simulink library "vmc"  (R2021b)
settings: Solver=VariableStepAuto  StartTime=0.0  StopTime=10.0  RelTol=1e-3
undefined symbols (not defined in the file or in its folder): AVMC_ACCDeltaTqIGain_X_kph, AVMC_ACCDeltaTqIGain_Y_mps2, AVMC_ACCDeltaTqIGainP2_X_kph, AVMC_ACCDeltaTqIGainP2_Y_mps2, AVMC_ACCDeltaTqPGain_X_kph, AVMC_ACCDeltaTqPGain_Y_kph, AVMC_ACCDeltaTqPGainP2_X_kph, AVMC_ACCDeltaTqPGainP2_Y_kph, AVMC_ACCLongSteadyCtrl_X_kph, AVMC_CCAccelCMD_X_kph, AVMC_CCAccelCMD_Y_kph, AVMC_CCDeltaTqIGain_X_kph, AVMC_CCDeltaTqIGain_Y_mps2, AVMC_CCDeltaTqPGain_X_kph, AVMC_CCDeltaTqPGain_Y_kph, AVMC_CCLongSteadyCtrl_X_kph, AVMC_DISCDeltaTqIGainP2_X_kph, AVMC_DISCDeltaTqIGainP2_Y_mps2, AVMC_ESCRegenOut_X_kph, AVMC_ESCRegenOut_Y_Deg, AVMC_ESCRegenOutEnSpd_X_Deg, AVMC_LatESCRegenOut_X_kph, AVMC_LatESCRegenOut_Y_Deg, AVMC_LongAccDeadZone_X_kph, AVMC_LongAccDeadZoneP2_X_kph, AVMC_LongAccFiltTs_X_Gps, AVMC_LongAccFiltTsP2_X_Gps, AVMC_MCPresBaseTq_X_bar, AVMC_MSAAccelCMD_X_kph, AVMC_MSAAccelCMD_Y_kph, AVMC_MSADeltaTqIGain_X_kph, AVMC_MSADeltaTqIGain_Y_mps2, AVMC_MSADeltaTqPGain_X_kph, AVMC_MSADeltaTqPGain_Y_kph, AVMC_MSALongSteadyCtrl_X_kph, AVMC_MSAPedalOvrd_X_kph, AVMC_MSASpdBand_X_kph, AVMC_OPDDisSlideRate_X_Deg, AVMC_RDCDetectTime_X_kph, AVMC_RDCDetectTime_Y_pct, AVMC_RDCEnSlideRate_X_Deg, AVMC_StESCYaw_X_kph, AVMC_StESCYaw_Y_Deg, AVMC_StESCYawCom_X_kph, AVMC_StESCYawCom_Y_Gps, AVMC_TMSpdBaseTq_X_rpm, C_TASK_10MS_S, C_TASK_5MS_S, DEG2RAD, Discrete, ENUM_ADASACCSTA_ACTIVE, ENUM_ADASACCSTA_OVERRIDE, ENUM_ADASACCSTA_STANDBY, ENUM_ADASMSASTA_ACTIVE, ENUM_ADASMSASTA_ERROR, ENUM_ADASMSASTA_OFF, ENUM_ADASMSASTA_OVERSPEED, ENUM_ADASMSASTA_STANDBY, ENUM_ADASMSASTA_UNDERSPEED, ENUM_ADASMSASTA_UNLIMIT ... (+254)
libraries: hcu_lib x57, simulink x49, ctrlSharedLib x6, simulink_extras x1
(part 6 of 9)

== system vmc/VMC/Slide Rate  Calculation/4Wheel Calculation ==
  VINP_LFRawWhlSpeed_kph : Inport
  VINP_RFRawWhlSpeed_kph : Inport  Port=2
  VINP_LRRawWhlSpeed_kph : Inport  Port=3
  VINP_RRRawWhlSpeed_kph : Inport  Port=4
  VVMC_LongAcc_Gps : Inport  Port=5
  task_time_s : Inport  Port=6
  VINP_VehSpeed_kph : Inport  Port=7
  VTQD_AfterAvailableTqDemFr_Nm : Inport  Port=8
  VTQD_AfterAvailableTqDemRr_Nm : Inport  Port=9
  VTQD_GearActualPosn_enum : Inport  Port=10
  VINP_LongAccel_Gps : Inport  Port=11
  VVMC_CalibratedAccX_G : Inport  Port=12
  Constant1 : Constant  Value=KVMC_SlideRateLongGSW_flg
  Constant3 : Constant  Value=KVMC_4WheelLongAccSW_flg
  Determination : Subsystem
  LF Wheel : Subsystem
  LR Wheel : Subsystem
  RF Wheel : Subsystem
  RR Wheel : Subsystem
  Switch : Switch  Criteria=u2 > Threshold
  Switch1 : Switch  Criteria=u2 > Threshold
  VVMC_LF4WhlSpdSlideRate_pct : Outport
  VVMC_RF4WhlSpdSlideRate_pct : Outport  Port=2
  VVMC_LR4WhlSpdSlideRate_pct : Outport  Port=3
  VVMC_RR4WhlSpdSlideRate_pct : Outport  Port=4
  VVMC_PredictVehSpd_kph : Outport  Port=5
  VVMC_4WhlSpdSlideRate_pct : Outport  Port=6
  VVMC_AllWhlSkid_flg : Outport  Port=7
  wires:
  [VVMC_4WhlSpdSlideRate_pct] -> VVMC_4WhlSpdSlideRate_pct/1
  [VVMC_PredictVehSpd_kph] -> VVMC_PredictVehSpd_kph/1
  VINP_VehSpeed_kph/1 -> [VINP_VehSpeed_kph]
  task_time_s/1 -> [task_time_s]
  [VVMC_LR4WhlSpdSlideRate_pct] -> VVMC_LR4WhlSpdSlideRate_pct/1
  [VVMC_RR4WhlSpdSlideRate_pct] -> VVMC_RR4WhlSpdSlideRate_pct/1
  [VVMC_RF4WhlSpdSlideRate_pct] -> VVMC_RF4WhlSpdSlideRate_pct/1
  [VVMC_LF4WhlSpdSlideRate_pct] -> VVMC_LF4WhlSpdSlideRate_pct/1
  VINP_LRRawWhlSpeed_kph/1 -> [VINP_LRRawWhlSpeed_kph]
  VINP_LFRawWhlSpeed_kph/1 -> [VINP_LFRawWhlSpeed_kph]
  VINP_RFRawWhlSpeed_kph/1 -> [VINP_RFRawWhlSpeed_kph]
  VINP_RRRawWhlSpeed_kph/1 -> [VINP_RRRawWhlSpeed_kph]
  [VVMC_AllWhlSkid_flg] -> VVMC_AllWhlSkid_flg/1
  VTQD_AfterAvailableTqDemFr_Nm/1 -> [VTQD_AfterAvailableTqDemFr_Nm]
  VTQD_AfterAvailableTqDemRr_Nm/1 -> [VTQD_AfterAvailableTqDemRr_Nm]
  VTQD_GearActualPosn_enum/1 -> [VTQD_GearActualPosn_enum]
  [VVMC_LRPreVehSpd_kph] -> Determination/17(VVMC_LRPreVehSpd_kph)
  [VVMC_4WheelLongAcc_Gps] -> LF Wheel/1(VVMC_4WheelLongAcc_Gps)
  [VINP_RRRawWhlSpeed_kph] -> RR Wheel/3(VINP_RRRawWhlSpeed_kph)
  [VINP_LRRawWhlSpeed_kph] -> LR Wheel/3(VINP_LRRawWhlSpeed_kph)
  [VINP_RFRawWhlSpeed_kph] -> RF Wheel/3(VINP_RFRawWhlSpeed_kph)
  [VTQD_GearActualPosn_enum] -> RF Wheel/4(VTQD_GearActualPosn_enum)
  LF Wheel/1(VVMC_LFPreVehSpd_kph) -> [VVMC_LFPreVehSpd_kph]
  RR Wheel/1(VVMC_RRPreVehSpd_kph) -> [VVMC_RRPreVehSpd_kph]
  [VTQD_GearActualPosn_enum] -> LR Wheel/4(VTQD_GearActualPosn_enum)
  [VVMC_LF4WhlSpdSlideRate_pct] -> Determination/9(VVMC_LF4WhlSpdSlideRate_pct)
  [VVMC_RRWhlSkid_flg] -> Determination/8(VVMC_RRWhlSkid_flg)
  [VINP_LFRawWhlSpeed_kph] -> LF Wheel/3(VINP_LFRawWhlSpeed_kph)
  [task_time_s] -> RR Wheel/2(task_time_s)
  [task_time_s] -> RF Wheel/2(task_time_s)
  [VVMC_RR4WhlSpdSlideRate_pct] -> Determination/12(VVMC_RR4WhlSpdSlideRate_pct)
  RR Wheel/3(VVMC_RR4WhlSpdSlideRate_pct) -> [VVMC_RR4WhlSpdSlideRate_pct]
  [VTQD_AfterAvailableTqDemFr_Nm] -> Determination/13(VTQD_AfterAvailableTqDemFr_Nm)
  [VVMC_LR4WhlSpdSlideRate_pct] -> Determination/11(VVMC_LR4WhlSpdSlideRate_pct)
  [VTQD_GearActualPosn_enum] -> Determination/4(VTQD_GearActualPosn_enum)
  [task_time_s] -> Determination/2(task_time_s)
  [VVMC_LFWhlSkid_flg] -> Determination/5(VVMC_LFWhlSkid_flg)
  [VINP_VehSpeed_kph] -> Determination/3(VINP_VehSpeed_kph)
  [VVMC_RRPreVehSpd_kph] -> Determination/18(VVMC_RRPreVehSpd_kph)
  Determination/2(VVMC_AllWhlSkid_flg) -> [VVMC_AllWhlSkid_flg]
  Determination/1(VVMC_PredictVehSpd_kph) -> [VVMC_PredictVehSpd_kph]
  Determination/3(VVMC_4WhlSpdSlideRate_pct) -> [VVMC_4WhlSpdSlideRate_pct]
  [VVMC_RFWhlSkid_flg] -> Determination/6(VVMC_RFWhlSkid_flg)
  LR Wheel/3(VVMC_LR4WhlSpdSlideRate_pct) -> [VVMC_LR4WhlSpdSlideRate_pct]
  LR Wheel/2(VVMC_LRWhlSkid_flg) -> [VVMC_LRWhlSkid_flg]
  [VVMC_LRWhlSkid_flg] -> Determination/7(VVMC_LRWhlSkid_flg)
  RF Wheel/1(VVMC_RFPreVehSpd_kph) -> [VVMC_RFPreVehSpd_kph]
  [task_time_s] -> LR Wheel/2(task_time_s)
  [VVMC_RFPreVehSpd_kph] -> Determination/16(VVMC_RFPreVehSpd_kph)
  LR Wheel/1(VVMC_LRPreVehSpd_kph) -> [VVMC_LRPreVehSpd_kph]
  [VVMC_4WheelLongAcc_Gps] -> RF Wheel/1(VVMC_4WheelLongAcc_Gps)
  RR Wheel/2(VVMC_RRWhlSkid_flg) -> [VVMC_RRWhlSkid_flg]
  [VVMC_LFPreVehSpd_kph] -> Determination/15(VVMC_LFPreVehSpd_kph)
  [VVMC_RF4WhlSpdSlideRate_pct] -> Determination/10(VVMC_RF4WhlSpdSlideRate_pct)
  [VTQD_AfterAvailableTqDemRr_Nm] -> Determination/14(VTQD_AfterAvailableTqDemRr_Nm)
  LF Wheel/2(VVMC_LFWhlSkid_flg) -> [VVMC_LFWhlSkid_flg]
  RF Wheel/2(VVMC_RFWhlSkid_flg) -> [VVMC_RFWhlSkid_flg]
  [VVMC_4WheelLongAcc_Gps] -> Determination/1(VVMC_4WheelLongAcc_Gps)
  [VVMC_4WheelLongAcc_Gps] -> RR Wheel/1(VVMC_4WheelLongAcc_Gps)
  [VTQD_GearActualPosn_enum] -> RR Wheel/4(VTQD_GearActualPosn_enum)
  [VVMC_4WheelLongAcc_Gps] -> LR Wheel/1(VVMC_4WheelLongAcc_Gps)
  RF Wheel/3(VVMC_RF4WhlSpdSlideRate_pct) -> [VVMC_RF4WhlSpdSlideRate_pct]
  LF Wheel/3(VVMC_LF4WhlSpdSlideRate_pct) -> [VVMC_LF4WhlSpdSlideRate_pct]
  [task_time_s] -> LF Wheel/2(task_time_s)
  [VTQD_GearActualPosn_enum] -> LF Wheel/4(VTQD_GearActualPosn_enum)
  Constant3/1 -> Switch/2
  Switch/1 -> [VVMC_4WheelLongAcc_Gps]  "VVMC_4WheelLongAcc_Gps"
  VINP_LongAccel_Gps/1 -> [VINP_LongAccel_Gps]
  VVMC_LongAcc_Gps/1 -> [VVMC_LongAcc_Gps]
  [VVMC_LongAcc_Gps] -> Switch/3
  Switch1/1 -> Switch/1
  [VINP_LongAccel_Gps] -> Switch1/3
  Constant1/1 -> Switch1/2
  [VVMC_CalibratedAccX_G] -> Switch1/1
  VVMC_CalibratedAccX_G/1 -> [VVMC_CalibratedAccX_G]

== system vmc/VMC/Slide Rate  Calculation/Alternative Wheel Slide Calculation ==
  VINP_LFRawWhlSpeed_kph : Inport
  VINP_RFRawWhlSpeed_kph : Inport  Port=2
  VINP_LRRawWhlSpeed_kph : Inport  Port=3
  VINP_RRRawWhlSpeed_kph : Inport  Port=4
  Abs : Abs
  Abs1 : Abs
  Add : Sum  Inputs=+-
  Add1 : Sum  Inputs=+-
  Constant{,3,5,8} (4 alike) : Constant  Value=KVMC_RawWhlSpeedDeadZone_kph
  Constant1 : Constant  Value=ONE_FLOAT
  Constant2 : Constant  Value=ONE_PERCENT
  Constant4 : Constant  Value=ZERO_FLOAT
  Constant6 : Constant  Value=ONE_FLOAT
  Constant7 : Constant  Value=ONE_PERCENT
  Constant9 : Constant  Value=ZERO_FLOAT
  Divide : Product  Inputs=*//
  Divide1 : Product  Inputs=*//
  Relational Operator{,1..3} (4 alike) : RelationalOperator  Operator=<=  OutDataTypeStr=boolean  RndMeth=Simplest
  Relational Operator4 : RelationalOperator  OutDataTypeStr=boolean  RndMeth=Simplest
  Switch{,1..4} (5 alike) : Switch  Criteria=u2 > Threshold
  VVMC_AltLWhlSlideRate_pct : Outport
  VVMC_AltRWhlSlideRate_pct : Outport  Port=2
  VVMC_AltWhlSlideRate_pct : Outport  Port=3
  wires:
  VINP_RRRawWhlSpeed_kph/1 -> [VINP_RRRawWhlSpeed_kph]
  Relational Operator1/1 -> Switch1/2
  Abs/1 -> Relational Operator4/1
  Divide/1 -> Switch1/3  "VVMC_CalAltLWhlSlideRate_pct"
  Constant1/1 -> Switch/1
  [VINP_LFRawWhlSpeed_kph] -> Add/2
  Switch1/1 -> [VVMC_AltLWhlSlideRate_pct]  "VVMC_AltLWhlSlideRate_pct"
  Constant6/1 -> Switch2/1
  Relational Operator3/1 -> Switch3/2
  Relational Operator4/1 -> Switch4/2
  [VVMC_AltLWhlSlideRate_pct] -> Abs/1
  [VVMC_AltLWhlSlideRate_pct] -> VVMC_AltLWhlSlideRate_pct/1
  VINP_LFRawWhlSpeed_kph/1 -> [VINP_LFRawWhlSpeed_kph]
  VINP_LRRawWhlSpeed_kph/1 -> [VINP_LRRawWhlSpeed_kph]
  VINP_RFRawWhlSpeed_kph/1 -> [VINP_RFRawWhlSpeed_kph]
  [VVMC_AltRWhlSlideRate_pct] -> Switch4/3
  Switch3/1 -> [VVMC_AltRWhlSlideRate_pct]  "VVMC_AltRWhlSlideRate_pct"
  Constant4/1 -> Switch1/1
  Constant3/1 -> Relational Operator1/2
  [VVMC_AltRWhlSlideRate_pct] -> Abs1/1
  [VVMC_AltLWhlSlideRate_pct] -> Switch4/1
  Switch4/1 -> [VVMC_AltWhlSlideRate_pct]  "VVMC_AltWhlSlideRate_pct"
  Constant2/1 -> Divide/2
  Constant7/1 -> Divide1/2
  Switch/1 -> Divide/3
  Constant9/1 -> Switch3/1
  [VINP_LFRawWhlSpeed_kph] -> Switch/3
  Relational Operator/1 -> Switch/2
  [VVMC_AltWhlSlideRate_pct] -> VVMC_AltWhlSlideRate_pct/1
  [VINP_RFRawWhlSpeed_kph] -> Add1/2
  Add/1 -> Divide/1
  Constant/1 -> Relational Operator/2
  [VINP_LFRawWhlSpeed_kph] -> Relational Operator1/1
  Abs1/1 -> Relational Operator4/2
  [VINP_RRRawWhlSpeed_kph] -> Add1/1
  [VINP_RFRawWhlSpeed_kph] -> Relational Operator3/1
  [VINP_RFRawWhlSpeed_kph] -> Switch2/3
  Add1/1 -> Divide1/1
  [VINP_LFRawWhlSpeed_kph] -> Relational Operator/1
  [VINP_LRRawWhlSpeed_kph] -> Add/1
  [VINP_RFRawWhlSpeed_kph] -> Relational Operator2/1
  Constant8/1 -> Relational Operator3/2
  Constant5/1 -> Relational Operator2/2
  Divide1/1 -> Switch3/3  "VVMC_CalAltRWhlSlideRate_pct"
  Switch2/1 -> Divide1/3
  Relational Operator2/1 -> Switch2/2
  [VVMC_AltRWhlSlideRate_pct] -> VVMC_AltRWhlSlideRate_pct/1

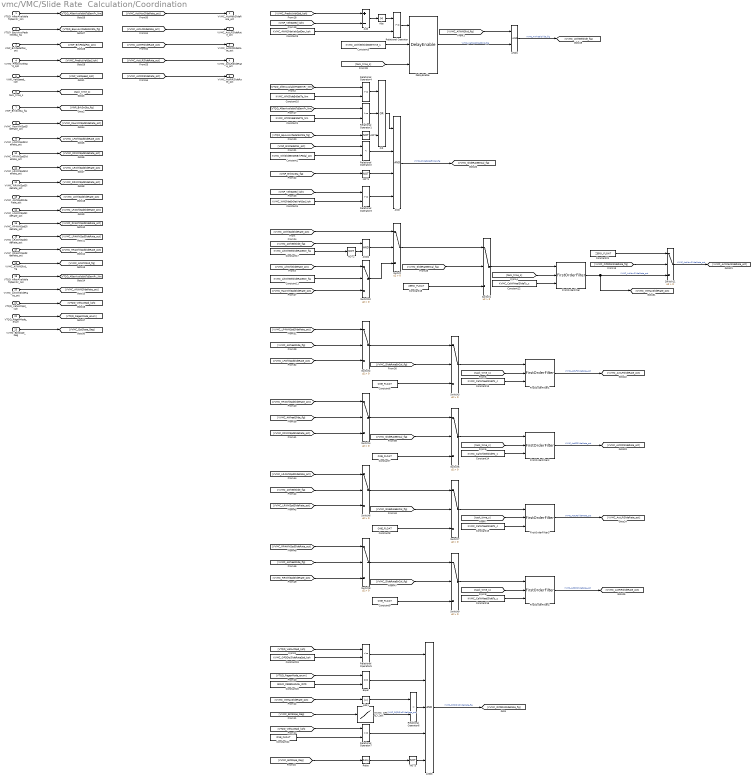
== system vmc/VMC/Slide Rate  Calculation/Coordination ==
  VTQD_AfterAvailableTqDemFr_Nm : Inport
  VTQD_EquivAccPedalSWSta_flg : Inport  Port=2
  VINP_BrkPedalPos_pct : Inport  Port=3
  VVMC_PredictVehSpd_kph : Inport  Port=4
  VINP_VehSpeed_kph : Inport  Port=5
  task_time_s : Inport  Port=6
  VINP_BrkSwSta_flg : Inport  Port=7
  VVMC_RawWhlSpdSlideRate_pct : Inport  Port=8
  VVMC_LFWhlSpdSlideRate_pct : Inport  Port=9
  VVMC_RFWhlSpdSlideRate_pct : Inport  Port=10
  VVMC_LRWhlSpdSlideRate_pct : Inport  Port=11
  VVMC_RRWhlSpdSlideRate_pct : Inport  Port=12
  VVMC_4WhlSpdSlideRate_pct : Inport  Port=13
  VVMC_LF4WhlSpdSlideRate_pct : Inport  Port=14
  VVMC_RF4WhlSpdSlideRate_pct : Inport  Port=15
  VVMC_LR4WhlSpdSlideRate_pct : Inport  Port=16
  VVMC_RR4WhlSpdSlideRate_pct : Inport  Port=17
  VVMC_AllWhlSkid_flg : Inport  Port=18
  VTQD_AfterAvailableTqDemRr_Nm : Inport  Port=19
  VVMC_AltWhlSlideRate_pct : Inport  Port=20
  VTQD_VehActSpd_kph : Inport  Port=21
  VTQD_RegenMode_enum : Inport  Port=22
  VVMC_EstSlope_Deg : Inport  Port=23
  AND : Logic  Inputs=4  AllPortsSameDT=off  OutDataTypeStr=boolean
  AND1 : Logic  AllPortsSameDT=off  OutDataTypeStr=boolean
  AND2 : Logic  AllPortsSameDT=off  OutDataTypeStr=boolean
  AND3 : Logic  Inputs=5  AllPortsSameDT=off  OutDataTypeStr=boolean
  Abs : Abs
  Abs1 : Abs
  Add : Sum  Inputs=+-
  Constant1 : Constant  Value=KVMC_WhlSlideEnDetTq_Nm
  Constant10 : Constant  Value=KVMC_WhlSlideEnDetTq_Nm
  Constant11 : Constant  Value=KVMC_AltWheelSlideRateSW_flg
  Constant{12..16} (5 alike) : Constant  Value=KVMC_CalWhleelSlideTs_c
  Constant17 : Constant  Value=KVMC_AltWheelSlideRateSW_flg
  Constant18 : Constant  Value=ZERO_FLOAT
  Constant19 : Constant  Value=KVMC_OPDDisSlideRateSpd_kph
  Constant2 : Constant  Value=KVMC_WhlSlideEnDetBrkPedal_pct
  Constant20 : Constant  Value=ENUM_REGENLEVEL_OPD
  Constant21 : Constant  Value=ZERO_FLOAT
  Constant{6..9,22} (5 alike) : Constant  Value=ONE_FLOAT
  Constant3 : Constant  Value=KVMC_4WhlSlideVehSpdDev_kph
  Constant4 : Constant  Value=KVMC_WhlSlideEnDetVehSpd_kph
  Constant5 : Constant  Value=KVMC_4WhleelSlideDetTime_s
  DelayEnable : hcu_lib/Basic_Blocks/DelayEnable
  Equal : RelationalOperator  Operator===  OutDataTypeStr=boolean  RndMeth=Simplest
  FirstOrderFilter{,1..4} (5 alike) : hcu_lib/Basic_Blocks/FirstOrderFilter
  MVMC_OPDDisSlideRate_Y_pct : Lookup_n-D  NumberOfTableDimensions=1  BreakpointsForDimension1=AVMC_OPDDisSlideRate_X_Deg  Table=MVMC_OPDDisSlideRate_Y_pct  InternalRulePriority=Speed  RndMeth=Simplest  InputSameDT=on
  NOT{,1..3} (4 alike) : Logic  Operator=NOT  AllPortsSameDT=off  OutDataTypeStr=boolean
  OR : Logic  Operator=OR  Inputs=3  AllPortsSameDT=off  OutDataTypeStr=boolean
  Relational Operator{,1,3..4,7} (5 alike) : RelationalOperator  OutDataTypeStr=boolean  RndMeth=Simplest
  Relational Operator2 : RelationalOperator  Operator=<  OutDataTypeStr=boolean  RndMeth=Simplest
  Relational Operator5 : RelationalOperator  Operator=<=  OutDataTypeStr=boolean  RndMeth=Simplest
  Relational Operator6 : RelationalOperator  Operator=<  OutDataTypeStr=boolean  RndMeth=Simplest
  Relay : Relay  OnSwitchValue=KTQD_OPDHoldGradeUp_Deg  OffSwitchValue=KTQD_OPDHoldGradeDown_Deg  OutDataTypeStr=boolean
  Switch{,1..11} (12 alike) : Switch  Criteria=u2 > Threshold
  VVMC_ActMaxSlideRate_pct : Outport
  VVMC_ActLFSlideRate_pct : Outport  Port=2
  VVMC_ActRFSlideRate_pct : Outport  Port=3
  VVMC_ActLRSlideRate_pct : Outport  Port=4
  VVMC_ActRRSlideRate_pct : Outport  Port=5
  wires:
  VVMC_RR4WhlSpdSlideRate_pct/1 -> [VVMC_RR4WhlSpdSlideRate_pct]
  VVMC_LR4WhlSpdSlideRate_pct/1 -> [VVMC_LR4WhlSpdSlideRate_pct]
  VVMC_RF4WhlSpdSlideRate_pct/1 -> [VVMC_RF4WhlSpdSlideRate_pct]
  VVMC_LF4WhlSpdSlideRate_pct/1 -> [VVMC_LF4WhlSpdSlideRate_pct]
  VVMC_4WhlSpdSlideRate_pct/1 -> [VVMC_4WhlSpdSlideRate_pct]
  VVMC_LRWhlSpdSlideRate_pct/1 -> [VVMC_LRWhlSpdSlideRate_pct]
  VVMC_RRWhlSpdSlideRate_pct/1 -> [VVMC_RRWhlSpdSlideRate_pct]
  VVMC_LFWhlSpdSlideRate_pct/1 -> [VVMC_LFWhlSpdSlideRate_pct]
  VVMC_RFWhlSpdSlideRate_pct/1 -> [VVMC_RFWhlSpdSlideRate_pct]
  VVMC_RawWhlSpdSlideRate_pct/1 -> [VVMC_RawWhlSpdSlideRate_pct]
  task_time_s/1 -> [task_time_s]
  VINP_BrkSwSta_flg/1 -> [VINP_BrkSwSta_flg]
  VINP_VehSpeed_kph/1 -> [VINP_VehSpeed_kph]
  VINP_BrkPedalPos_pct/1 -> [VINP_BrkPedalPos_pct]
  VTQD_EquivAccPedalSWSta_flg/1 -> [VTQD_EquivAccPedalSWSta_flg]
  VTQD_AfterAvailableTqDemFr_Nm/1 -> [VTQD_AfterAvailableTqDemFr_Nm]
  VVMC_PredictVehSpd_kph/1 -> [VVMC_PredictVehSpd_kph]
  [VVMC_ActRFSlideRate_pct] -> VVMC_ActRFSlideRate_pct/1
  [VVMC_ActLFSlideRate_pct] -> VVMC_ActLFSlideRate_pct/1
  [VVMC_ActMaxSlideRate_pct] -> VVMC_ActMaxSlideRate_pct/1
  [VVMC_ActLRSlideRate_pct] -> VVMC_ActLRSlideRate_pct/1
  [VVMC_ActRRSlideRate_pct] -> VVMC_ActRRSlideRate_pct/1
  [VINP_VehSpeed_kph] -> Add/2
  OR/1 -> AND/1
  [VVMC_RRWhlSpdSlideRate_pct] -> Switch8/3
  Constant4/1 -> Relational Operator3/2
  [VVMC_4WheelSlide_flg] -> AND2/1
  [VVMC_4WhlSpdSlideRate_pct] -> Switch/1
  [VVMC_SlideRateEnCal_flg] -> Switch9/2
  [VVMC_4WheelSlide_flg] -> Switch6/2
  [VVMC_LR4WhlSpdSlideRate_pct] -> Switch6/1
  [VTQD_EquivAccPedalSWSta_flg] -> NOT/1
  Constant8/1 -> Switch7/3
  [VVMC_LF4WhlSpdSlideRate_pct] -> Switch2/1
  Abs/1 -> Relational Operator/1
  Switch8/1 -> Switch9/1
  [VVMC_LRWhlSpdSlideRate_pct] -> Switch6/3
  [VVMC_SlideRateEnCal_flg] -> Switch5/2
  Switch/1 -> Switch1/1
  Constant7/1 -> Switch5/3
  Switch4/1 -> Switch5/1
  Constant9/1 -> Switch9/3
  Constant5/1 -> DelayEnable/2
  [VINP_BrkPedalPos_pct] -> Relational Operator2/1
  Switch6/1 -> Switch7/1
  NOT1/1 -> AND/3
  [VVMC_RFWhlSpdSlideRate_pct] -> Switch4/3
  [VVMC_SlideRateEnCal_flg] -> Switch3/2
  Constant18/1 -> Switch1/3
  Constant6/1 -> Switch3/3
  Switch2/1 -> Switch3/1
  [VVMC_RF4WhlSpdSlideRate_pct] -> Switch4/1
  [VVMC_4WheelSlide_flg] -> Switch4/2
  Add/1 -> Abs/1
  [VVMC_4WheelSlide_flg] -> Switch2/2
  Relational Operator/1 -> DelayEnable/1
  [VVMC_4WheelSlide_flg] -> Switch8/2
  [VVMC_RR4WhlSpdSlideRate_pct] -> Switch8/1
  Relational Operator3/1 -> AND/4
  [VVMC_LFWhlSpdSlideRate_pct] -> Switch2/3
  Constant1/1 -> Relational Operator1/2
  [VVMC_PredictVehSpd_kph] -> Add/1
  [VINP_BrkSwSta_flg] -> NOT1/1
  [VINP_VehSpeed_kph] -> Relational Operator3/1
  Relational Operator2/1 -> AND/2
  AND/1 -> [VVMC_SlideRateEnCal_flg]  "VVMC_SlideRateEnCal_flg"
  [VVMC_SlideRateEnCal_flg] -> Switch7/2
  Constant3/1 -> Relational Operator/2
  Constant2/1 -> Relational Operator2/2
  [task_time_s] -> DelayEnable/3
  VVMC_AllWhlSkid_flg/1 -> [VVMC_AllWhlSkid_flg]
  DelayEnable/1 -> AND1/2  "VVMC_VehSpdPredSkid_flg"
  AND1/1 -> [VVMC_4WheelSlide_flg]  "VVMC_4WheelSlide_flg"
  [VVMC_AllWhlSkid_flg] -> AND1/1
  Constant10/1 -> Relational Operator4/2
  [VTQD_AfterAvailableTqDemRr_Nm] -> Relational Operator4/1
  NOT/1 -> OR/3
  Relational Operator1/1 -> OR/2
  Relational Operator4/1 -> OR/1
  [VTQD_AfterAvailableTqDemFr_Nm] -> Relational Operator1/1
  VTQD_AfterAvailableTqDemRr_Nm/1 -> [VTQD_AfterAvailableTqDemRr_Nm]
  VVMC_AltWhlSlideRate_pct/1 -> [VVMC_AltWhlSlideRate_pct]
  [VVMC_RawWhlSpdSlideRate_pct] -> Switch10/3
  Switch10/1 -> Switch/3
  [VVMC_AltWhlSlideRate_pct] -> Switch10/1
  Constant11/1 -> Switch10/2
  Switch1/1 -> FirstOrderFilter/1
  FirstOrderFilter1/1 -> [VVMC_ActLFSlideRate_pct]  "VVMC_ActLFSlideRate_pct"
  Switch3/1 -> FirstOrderFilter1/1
  Switch5/1 -> FirstOrderFilter2/1
  FirstOrderFilter2/1 -> [VVMC_ActRFSlideRate_pct]  "VVMC_ActRFSlideRate_pct"
  Switch7/1 -> FirstOrderFilter3/1
  FirstOrderFilter3/1 -> [VVMC_ActLRSlideRate_pct]  "VVMC_ActLRSlideRate_pct"
  Switch9/1 -> FirstOrderFilter4/1
  FirstOrderFilter4/1 -> [VVMC_ActRRSlideRate_pct]  "VVMC_ActRRSlideRate_pct"
  Constant12/1 -> FirstOrderFilter/3
  [task_time_s] -> FirstOrderFilter/2
  [task_time_s] -> FirstOrderFilter1/2
  Constant13/1 -> FirstOrderFilter1/3
  [task_time_s] -> FirstOrderFilter2/2
  Constant14/1 -> FirstOrderFilter2/3
  Constant15/1 -> FirstOrderFilter3/3
  [task_time_s] -> FirstOrderFilter3/2
  Constant16/1 -> FirstOrderFilter4/3
  [task_time_s] -> FirstOrderFilter4/2
  Constant17/1 -> NOT2/1
  NOT2/1 -> AND2/2
  AND2/1 -> Switch/2
  VVMC_EstSlope_Deg/1 -> [VVMC_EstSlope_Deg]
  VTQD_RegenMode_enum/1 -> [VTQD_RegenMode_enum]
  VTQD_VehActSpd_kph/1 -> [VTQD_VehActSpd_kph]
  [VTQD_VehActSpd_kph] -> Relational Operator5/1
  Constant19/1 -> Relational Operator5/2
  [VTQD_RegenMode_enum] -> Equal/1
  Constant20/1 -> Equal/2
  [VVMC_EstSlope_Deg] -> MVMC_OPDDisSlideRate_Y_pct/1
  MVMC_OPDDisSlideRate_Y_pct/1 -> Relational Operator6/2  "VVMC_OPDDisSlideRate_pct"
  Relational Operator5/1 -> AND3/1
  Equal/1 -> AND3/2
  Relational Operator6/1 -> AND3/3
  AND3/1 -> [VVMC_OPDDisSlideRate_flg]  "VVMC_OPDDisSlideRate_flg"
  [VVMC_IntMaxSlideRate_pct] -> Abs1/1
  Abs1/1 -> Relational Operator6/1
  [VVMC_SlideRateEnCal_flg] -> Switch1/2
  FirstOrderFilter/1 -> [VVMC_IntMaxSlideRate_pct], Switch11/3  "VVMC_IntMaxSlideRate_pct"
  Switch11/1 -> [VVMC_ActMaxSlideRate_pct]  "VVMC_ActMaxSlideRate_pct"
  [VVMC_OPDDisSlideRate_flg] -> Switch11/2
  Constant21/1 -> Switch11/1
  Constant22/1 -> Relational Operator7/2
  [VTQD_VehActSpd_kph] -> Relational Operator7/1
  Relational Operator7/1 -> AND3/4
  NOT3/1 -> AND3/5
  Relay/1 -> NOT3/1
  [VVMC_EstSlope_Deg] -> Relay/1

== system vmc/VMC/Slide Rate  Calculation/Partial Wheel Calculation ==
  VINP_LFRawWhlSpeed_kph : Inport
  VINP_RFRawWhlSpeed_kph : Inport  Port=2
  VINP_LRRawWhlSpeed_kph : Inport  Port=3
  VINP_RRRawWhlSpeed_kph : Inport  Port=4
  VTQD_AfterAvailableTqDemFr_Nm : Inport  Port=5
  VTQD_AfterAvailableTqDemRr_Nm : Inport  Port=6
  Add{,1..4} (5 alike) : Sum  Inputs=+-
  Add5 : Sum
  Constant{,3,5,8,10,13,15,18,20,23} (10 alike) : Constant  Value=KVMC_RawWhlSpeedDeadZone_kph
  Constant{1,6,11,16,21,26} (6 alike) : Constant  Value=ONE_FLOAT
  Constant{2,7,12,17,22} (5 alike) : Constant  Value=ONE_PERCENT
  Constant{4,9,14,19,24..25} (6 alike) : Constant  Value=ZERO_FLOAT
  Constant27 : Constant  Value=MINUSONE_FLOAT
  Divide{,1..4} (5 alike) : Product  Inputs=*//
  Max : MinMax  Function=max  Inputs=4
  Max1 : MinMax  Inputs=4
  Product : Product
  Relational Operator{,1..10} (11 alike) : RelationalOperator  Operator=<=  OutDataTypeStr=boolean  RndMeth=Simplest
  Switch{,1..10} (11 alike) : Switch  Criteria=u2 > Threshold
  VVMC_RawWhlSpdSlideRate_pct : Outport
  VVMC_LFWhlSpdSlideRate_pct : Outport  Port=2
  VVMC_RFWhlSpdSlideRate_pct : Outport  Port=3
  VVMC_LRWhlSpdSlideRate_pct : Outport  Port=4
  VVMC_RRWhlSpdSlideRate_pct : Outport  Port=5
  wires:
  [VVMC_RRWhlSpdSlideRate_pct] -> VVMC_RRWhlSpdSlideRate_pct/1
  [VVMC_LRWhlSpdSlideRate_pct] -> VVMC_LRWhlSpdSlideRate_pct/1
  [VVMC_LFWhlSpdSlideRate_pct] -> VVMC_LFWhlSpdSlideRate_pct/1
  [VVMC_RFWhlSpdSlideRate_pct] -> VVMC_RFWhlSpdSlideRate_pct/1
  [VVMC_RawWhlSpdSlideRate_pct] -> VVMC_RawWhlSpdSlideRate_pct/1
  VINP_RRRawWhlSpeed_kph/1 -> [VINP_RRRawWhlSpeed_kph]
  VINP_LRRawWhlSpeed_kph/1 -> [VINP_LRRawWhlSpeed_kph]
  VINP_RFRawWhlSpeed_kph/1 -> [VINP_RFRawWhlSpeed_kph]
  VINP_LFRawWhlSpeed_kph/1 -> [VINP_LFRawWhlSpeed_kph]
  Constant15/1 -> Relational Operator6/2
  Relational Operator6/1 -> Switch6/2
  Constant16/1 -> Switch6/1
  Constant17/1 -> Divide3/2
  Switch6/1 -> Divide3/3
  Switch7/1 -> [VVMC_LRWhlSpdSlideRate_pct]  "VVMC_LRWhlSpdSlideRate_pct"
  Relational Operator7/1 -> Switch7/2
  [VINP_LRRawWhlSpeed_kph] -> Relational Operator7/1
  Constant18/1 -> Relational Operator7/2
  [VVMC_MinRawWhlSpeed_kph] -> Switch6/3
  [VVMC_MinRawWhlSpeed_kph] -> Relational Operator6/1
  [VINP_LRRawWhlSpeed_kph] -> Add3/1
  Add3/1 -> Divide3/1
  [VVMC_MinRawWhlSpeed_kph] -> Add3/2
  [VINP_RFRawWhlSpeed_kph] -> Max1/2
  [VINP_LRRawWhlSpeed_kph] -> Max1/3
  Max1/1 -> [VVMC_MinRawWhlSpeed_kph]  "VVMC_MinRawWhlSpeed_kph"
  Add/1 -> Divide/1
  Divide1/1 -> Switch3/3  "VVMC_LFCalWhlSpdSlideRate_pct"
  [VINP_LFRawWhlSpeed_kph] -> Relational Operator3/1
  Switch3/1 -> [VVMC_LFWhlSpdSlideRate_pct]  "VVMC_LFWhlSpdSlideRate_pct"
  Constant8/1 -> Relational Operator3/2
  Constant7/1 -> Divide1/2
  Product/1 -> [VVMC_RawWhlSpdSlideRate_pct]  "VVMC_RawWhlSpdSlideRate_pct"
  Constant2/1 -> Divide/2
  Relational Operator3/1 -> Switch3/2
  [VINP_RRRawWhlSpeed_kph] -> Relational Operator9/1
  [VVMC_MinRawWhlSpeed_kph] -> Switch/3
  Add4/1 -> Divide4/1
  Constant24/1 -> Switch9/1
  [VINP_LFRawWhlSpeed_kph] -> Max/1
  [VINP_RRRawWhlSpeed_kph] -> Max/4
  Constant14/1 -> Switch5/1
  Constant9/1 -> Switch3/1
  Constant21/1 -> Switch8/1
  Constant22/1 -> Divide4/2
  Switch4/1 -> Divide2/3
  Constant12/1 -> Divide2/2
  Divide3/1 -> Switch7/3  "VVMC_LRCalWhlSpdSlideRate_pct"
  Constant11/1 -> Switch4/1
  [VINP_RFRawWhlSpeed_kph] -> Add2/1
  [VINP_RFRawWhlSpeed_kph] -> Max/2
  Relational Operator4/1 -> Switch4/2
  Add2/1 -> Divide2/1
  [VVMC_MinRawWhlSpeed_kph] -> Add2/2
  [VVMC_MaxRawWhlSpeed_kph] -> Add/1
  [VINP_LRRawWhlSpeed_kph] -> Max/3
  [VVMC_MinRawWhlSpeed_kph] -> Relational Operator4/1
  Relational Operator1/1 -> Switch1/2
  Switch2/1 -> Divide1/3
  Divide2/1 -> Switch5/3  "VVMC_RFCalWhlSpdSlideRate_pct"
  [VINP_RRRawWhlSpeed_kph] -> Max1/4
  [VVMC_MinRawWhlSpeed_kph] -> Switch4/3
  Constant6/1 -> Switch2/1
  Max/1 -> [VVMC_MaxRawWhlSpeed_kph]  "VVMC_MaxRawWhlSpeed_kph"
  Constant19/1 -> Switch7/1
  [VINP_LFRawWhlSpeed_kph] -> Max1/1
  [VVMC_MinRawWhlSpeed_kph] -> Switch2/3
  [VINP_LFRawWhlSpeed_kph] -> Add1/1
  Constant13/1 -> Relational Operator5/2
  Constant23/1 -> Relational Operator9/2
  Add1/1 -> Divide1/1
  Constant3/1 -> Relational Operator1/2
  [VINP_RRRawWhlSpeed_kph] -> Add4/1
  Relational Operator2/1 -> Switch2/2
  Switch9/1 -> [VVMC_RRWhlSpdSlideRate_pct]  "VVMC_RRWhlSpdSlideRate_pct"
  [VVMC_MinRawWhlSpeed_kph] -> Switch8/3
  [VINP_RFRawWhlSpeed_kph] -> Relational Operator5/1
  [VVMC_MinRawWhlSpeed_kph] -> Relational Operator2/1
  Constant10/1 -> Relational Operator4/2
  Constant/1 -> Relational Operator/2
  Divide4/1 -> Switch9/3  "VVMC_RRCalWhlSpdSlideRate_pct"
  Relational Operator/1 -> Switch/2
  [VVMC_MaxRawWhlSpeed_kph] -> Relational Operator1/1
  [VVMC_MinRawWhlSpeed_kph] -> Add1/2
  [VVMC_MinRawWhlSpeed_kph] -> Add4/2
  Constant1/1 -> Switch/1
  Constant20/1 -> Relational Operator8/2
  Relational Operator9/1 -> Switch9/2
  Switch/1 -> Divide/3
  Switch8/1 -> Divide4/3
  Constant4/1 -> Switch1/1
  Switch5/1 -> [VVMC_RFWhlSpdSlideRate_pct]  "VVMC_RFWhlSpdSlideRate_pct"
  [VVMC_MinRawWhlSpeed_kph] -> Add/2
  Relational Operator5/1 -> Switch5/2
  Relational Operator8/1 -> Switch8/2
  Divide/1 -> Switch1/3  "VVMC_RawCalWhlSpdSlideRate_pct"
  Constant5/1 -> Relational Operator2/2
  [VVMC_MinRawWhlSpeed_kph] -> Relational Operator/1
  [VVMC_MinRawWhlSpeed_kph] -> Relational Operator8/1
  VTQD_AfterAvailableTqDemFr_Nm/1 -> [VTQD_AfterAvailableTqDemFr_Nm]
  VTQD_AfterAvailableTqDemRr_Nm/1 -> [VTQD_AfterAvailableTqDemRr_Nm]
  Relational Operator10/1 -> Switch10/2
  Constant27/1 -> Switch10/1
  [VTQD_AfterAvailableTqDemRr_Nm] -> Add5/2
  [VTQD_AfterAvailableTqDemFr_Nm] -> Add5/1
  Add5/1 -> Relational Operator10/1
  Constant26/1 -> Switch10/3
  Constant25/1 -> Relational Operator10/2
  Switch1/1 -> Product/2
  Switch10/1 -> Product/1

== system vmc/VMC/Subsystem1/Triggered Subsystem2 ==
  In1 : Inport
  Trigger : TriggerPort  VariantControl=(inherit)
  Out1 : Outport
  wires:
  In1/1 -> Out1/1

== system vmc/VMC/Subsystem1/Triggered Subsystem3 ==
  In1 : Inport
  Trigger : TriggerPort  VariantControl=(inherit)
  Out1 : Outport
  wires:
  In1/1 -> Out1/1
